simulink model "P2001_230206_CumulativeCostEM1"  (R2022b)
settings: Solver=VariableStepAuto  StartTime=0.0  StopTime=30  RelTol=1e-7
settings Model: Creator=turib  LastModifiedBy=turib
settings HardwareCC: ProdHWDeviceType=AMD->x86-64 (Windows64)

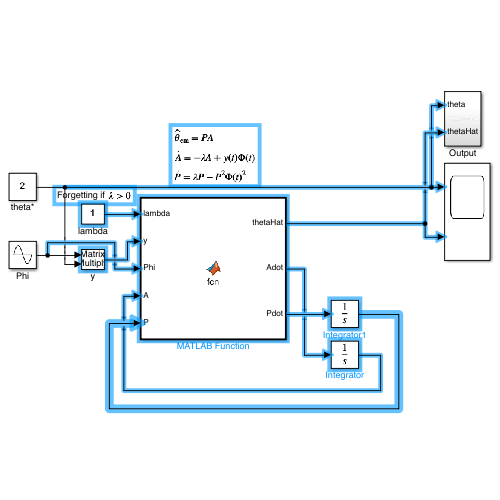
[thumbnail: Simulink's stored preview of the top-level diagram]
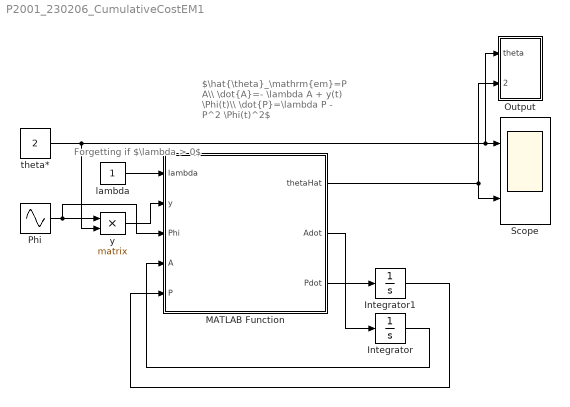
== system P2001_230206_CumulativeCostEM1 ==
  note: Forgetting if $\lambda > 0$
  note: $\hat{\theta}_\mathrm{em}=P A\\ \dot{A}=- \lambda A + y(t) \Phi(t)\\ \dot{P}=\lambda P - P^2 \Phi(t)^2$
  Integrator : Integrator  InitialCondition=1
  Integrator1 : Integrator  InitialCondition=1
  MATLAB Function : MATLAB Function  TreatAsAtomicUnit=on
  Output : Subsystem
  Phi : Sin  Frequency=2  Phase=1  SampleTime=0
  Scope : Scope  NumInputPorts=2
  lambda : Constant
  theta* : Constant  Value=2
  y : Product  Multiplication=Matrix(*)  OutDataTypeStr=double
  wires:
  theta*/1 -> Output/1(theta), Scope/1, y/2
  y/1 -> MATLAB Function/2(y)
  Phi/1 -> MATLAB Function/3(Phi), y/1
  MATLAB Function/2(Adot) -> Integrator/1
  MATLAB Function/1(thetaHat) -> Output/2(thetaHat), Scope/2
  lambda/1 -> MATLAB Function/1(lambda)
  MATLAB Function/3(Pdot) -> Integrator1/1
  Integrator1/1 -> MATLAB Function/5(P)
  Integrator/1 -> MATLAB Function/4(A)

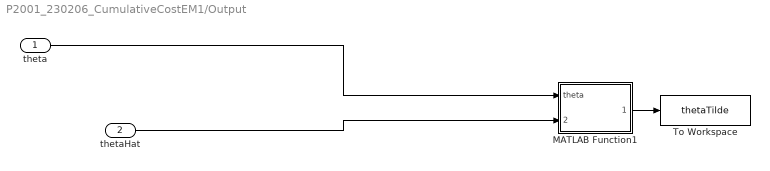
== system P2001_230206_CumulativeCostEM1/Output ==
  theta : Inport
  thetaHat : Inport  Port=2
  MATLAB Function1 : MATLAB Function  TreatAsAtomicUnit=on
  To Workspace : ToWorkspace  VariableName=thetaTilde  SampleTime=-1
  wires:
  MATLAB Function1/1(thetaTilde) -> To Workspace/1
  thetaHat/1 -> MATLAB Function1/2(thetaHat)
  theta/1 -> MATLAB Function1/1(theta)

== matlab function P2001_230206_CumulativeCostEM1/Output/MATLAB Function1 ==
  data: theta input; thetaTilde output; thetaHat input
function thetaTilde = error(theta, thetaHat)

thetaTilde = thetaHat - theta;

end

== matlab function P2001_230206_CumulativeCostEM1/MATLAB Function ==
  data: thetaHat output; lambda input; Adot output; y input; Phi input; A input; P input; Pdot output
function [thetaHat, Adot, Pdot] = fcn(lambda, y, Phi, ...
    A, P)

thetaHat = P * A;
Adot = - lambda * A + y * Phi;
Pdot = lambda * P - P ^ 2 * Phi ^ 2;
% B = inv(P);
% Jder = -2 * (A - B * thetaHat);

end
